simulink library "mbd_s32k1xx_ec_toolbox"  (Simulink 9.0)
settings: Solver=FixedStepDiscrete  StartTime=0.0  StopTime=10.0  FixedStep=0.1  RelTol=1e-3  EnableMultiTasking=on
InitFcn:
  | mbd_s32k_consistency_checks(bdroot(gcs));
(part 2 of 8)

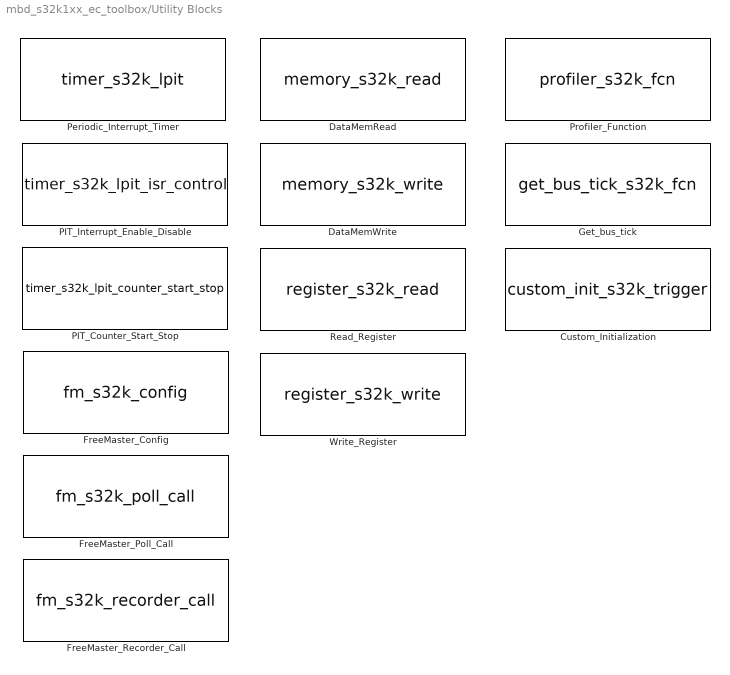
== system mbd_s32k1xx_ec_toolbox/Utility Blocks ==
  Custom_Initialization : S-Function  FunctionName=custom_init_s32k_trigger  SFunctionDeploymentMode=off  EnableBusSupport=off  mask(custom_init_s32k_trigger_block){}
      mask help: This block allows user to insert custom initialization code
      settings: NameChangeFcn=mbd_s12zvc_name_check(gcb);
      mask Help: web(fullfile(mbd_s32k_block_help, 'custom_init', 'custom_init_trigger.html'));
      mask Display:
      | disp('Initialization Call Insertion');
      | port_label('output', 1, 'Trigger');
      | image('nxp_logo.png', 'top-right');
  DataMemRead : S-Function  FunctionName=memory_s32k_read  Parameters=ptr_type  SFunctionDeploymentMode=off  EnableBusSupport=off  mask(memory_s32k_read){base=0x20000000, offset=0x0000, ptr=uint32_t}
      mask prompts: base "Address"; ptr "Pointer type"
      mask help: This block allows a direct memory read from the specified memory location.
      mask init:
      | [maskStr, ptr_type] = mbd_s32k_mem_init();
      settings: NameChangeFcn=mbd_s32k_name_check(gcb);
      mask Help: web(fullfile(mbd_s32k_block_help, 'memory', 'memory_read.html'));
      mask Callback base:
      | str = get_param(gcb, 'base');
      | len = length(str);
      | size = 8;
      | 
      | if (len > 2)
      |     if (strcmp(str(1:2), '0x'))
      |         str = str(3:len);
      |     end
      | end
      | %check if str is a valid hex number. if not, make a valid hex
      | isAllHex = all(isstrprop(str, 'xdigit'));
      | if (~isAllHex)
      |         str = dec2hex(0,size);
      |         len = length(str);
      | end
      | %get address from string
      | value = hex2dec(str);
      | 
      | %check range
      | if (value < 0)
      |     value = 0;
      | elseif (value > hex2dec('FFFF0000'))
      |     value = hex2dec('FFFF0000');
      | end
      | 
      | set_param(gcb, 'base', strcat('0x',dec2hex(value,size)));
      mask Callback offset:
      | str = get_param(gcb, 'offset');
      | len = length(str);
      | size = 4;
      | 
      | if (len > 2)
      |     if (strcmp(str(1:2), '0x'))
      |         str = str(3:len);
      |     end
      | end
      | %check if str is a valid hex number. if not, make a valid hex
      | isAllHex = all(isstrprop(str, 'xdigit'));
      | if (~isAllHex)
      |         str = dec2hex(0,size);
      |         len = length(str);
      | end
      | %get address from string
      | value = hex2dec(str);
      | 
      | %check range
      | if (value < 0)
      |     value = 0;
      | elseif (value > hex2dec('FFFF'))
      |     value = hex2dec('FFFF');
      | end
      | 
      | set_param(gcb, 'offset', strcat('0x',dec2hex(value,size)));
      mask TypeOptions ptr: uint8_t | uint16_t | uint32_t
      mask Display:
      | image('nxp_logo.png', 'top-right');
      | port_label('output',1,'Output');
      | 
      | disp(maskStr);
  DataMemWrite : S-Function  FunctionName=memory_s32k_write  Parameters=ptr_type  SFunctionDeploymentMode=off  EnableBusSupport=off  mask(memory_s32k_write){base=0x20000000, offset=0x0000, ptr=uint32_t}
      mask prompts: base "Address"; ptr "Pointer type"
      mask help: This block allows a direct write to the specified memory location.
      mask init:
      | [maskStr, ptr_type] = mbd_s32k_mem_init();
      settings: NameChangeFcn=mbd_s32k_name_check(gcb);
      mask Help: web(fullfile(mbd_s32k_block_help, 'memory', 'memory_write.html'));
      mask Callback base:
      | str = get_param(gcb, 'base');
      | len = length(str);
      | size = 8;
      | 
      | if (len > 2)
      |     if (strcmp(str(1:2), '0x'))
      |         str = str(3:len);
      |     end
      | end
      | %check if str is a valid hex number. if not, make a valid hex
      | isAllHex = all(isstrprop(str, 'xdigit'));
      | if (~isAllHex)
      |         str = dec2hex(0,size);
      |         len = length(str);
      | end
      | %get address from string
      | value = hex2dec(str);
      | 
      | %check range
      | if (value < 0)
      |     value = 0;
      | elseif (value > hex2dec('FFFF0000'))
      |     value = hex2dec('FFFF0000');
      | end
      | 
      | set_param(gcb, 'base', strcat('0x',dec2hex(value,size)));
      mask Callback offset:
      | str = get_param(gcb, 'offset');
      | len = length(str);
      | size = 4;
      | 
      | if (len > 2)
      |     if (strcmp(str(1:2), '0x'))
      |         str = str(3:len);
      |     end
      | end
      | %check if str is a valid hex number. if not, make a valid hex
      | isAllHex = all(isstrprop(str, 'xdigit'));
      | if (~isAllHex)
      |         str = dec2hex(0,size);
      |         len = length(str);
      | end
      | %get address from string
      | value = hex2dec(str);
      | 
      | %check range
      | if (value < 0)
      |     value = 0;
      | elseif (value > hex2dec('FFFF'))
      |     value = hex2dec('FFFF');
      | end
      | 
      | set_param(gcb, 'offset', strcat('0x',dec2hex(value,size)));
      mask TypeOptions ptr: uint8_t | uint16_t | uint32_t
      mask Display:
      | image('nxp_logo.png', 'top-right');
      | port_label('input',1,'Input');
      | 
      | disp(maskStr);
  FreeMaster_Config : S-Function  FunctionName=fm_s32k_config  Parameters=sFuncParams  SFunctionDeploymentMode=off  EnableBusSupport=off  mask(fm_s32k_config){interface=LPUART1, baudrate=19200, rxd=PTC6: [LPUART1_RX | Receive], txd=PTC7: [LPUART1_TX | Transmit], mode=Poll-driven, isr_prio=15, show_adv_opts=off, use_scope=on, max_scope_vars=8, use_recorder=on, max_rec_vars=8, rec_buff_size=1024, rec_timebase=0, rec_timebase_unit=seconds, comm_buffer_size_auto=on, comm_buffer_size=255, comm_rqueue_size_default=on, comm_rqueue_size=32}
      mask prompts: baudrate "Baud Rate"; rxd "RxD pin"; txd "TxD pin"; isr_prio "ISR Priority"; show_adv_opts "Show Advanced Options"; use_scope "Use Scope"; max_scope_vars "Max Variables"; use_recorder "Use Reccorder"; max_rec_vars "Max Variables"; rec_buff_size "Buffer size (0 - 65536)"; rec_timebase "Timebase (0 - 16384)"; comm_buffer_size_auto "Automatic buffer size"; comm_buffer_size "Buffer size (1-255)"; comm_rqueue_size_default "Default FIFO receiver queue size"; comm_rqueue_size "FIFO receiver queue size (1 - 255)"
      mask help: This block allows the user to configure the FreeMaster embedded-side software driver.
      mask init:
      | mbd_s32k_fm_config_init;
      | mbd_s32k_fm_display_instances;
      settings: NameChangeFcn=mbd_s32k_name_check(gcb);
      mask Help: web(fullfile(mbd_s32k_block_help, 'fm', 'fm_config.html'));
      mask TypeOptions interface: LPUART0 | LPUART1 | LPUART2 | CAN0 | CAN1 | CAN2
      mask Callback interface:
      | mbd_s32k_fm_config_cbk('interface');
      | mbd_s32k_fm_display_instances();
      mask TypeOptions baudrate: 1200 | 2400 | 4800 | 9600 | 14400 | 19200 | 38400 | 56000 | 57600 | 115200 | 128000 | 256000
      mask TypeOptions rxd: PTA19: [LPUART1_RX | Receive] | PTB23: [LPUART1_RX | Receive] | PTC6: [LPUART1_RX | Receive] | PTC8: [LPUART1_RX | Receive] | PTD13: [LPUART1_RX | Receive]
      mask TypeOptions txd: PTA18: [LPUART1_TX | Transmit] | PTB22: [LPUART1_TX | Transmit] | PTC7: [LPUART1_TX | Transmit] | PTC9: [LPUART1_TX | Transmit] | PTD14: [LPUART1_TX | Transmit]
      mask TypeOptions mode: Long Interrupt | Short Interrupt | Poll-driven
      mask Callback mode: mbd_s32k_fm_config_cbk('mode')
      mask TypeOptions isr_prio: 0 | 1 | 2 | 3 | 4 | 5 | 6 | 7 | 8 | 9 | 10 | 11 | 12 | 13 | 14 | 15
      mask Callback show_adv_opts: mbd_s32k_fm_config_cbk('show_adv_opts')
      mask Callback use_scope: mbd_s32k_fm_config_cbk('use_scope')
      mask TypeOptions max_scope_vars: 2 | 3 | 4 | 5 | 6 | 7 | 8
      mask Callback use_recorder: mbd_s32k_fm_config_cbk('use_recorder')
      mask TypeOptions max_rec_vars: 2 | 3 | 4 | 5 | 6 | 7 | 8
      mask TypeOptions rec_timebase_unit: seconds | milliseconds | microseconds | nanoseconds
      mask Callback comm_buffer_size_auto: mbd_s32k_fm_config_cbk('comm_buffer_size_auto')
      mask Callback comm_rqueue_size_default: mbd_s32k_fm_config_cbk('comm_rqueue_size_default')
      mask Display:
      | image('nxp_logo.png', 'top-right');
      | disp(maskStr)
  FreeMaster_Poll_Call : S-Function  FunctionName=fm_s32k_poll_call  SFunctionDeploymentMode=off  EnableBusSupport=off  mask(fm_s32k_poll_call){}
      mask help: This block allows the user to call the FMSTR_Call function in other places then main loop. The FMSTR_Call is placed in the main application loop when this block is not used.
      settings: NameChangeFcn=mbd_s32k_name_check(gcb);
      mask Help: web(fullfile(mbd_s32k_block_help, 'fm', 'fm_poll_call.html'));
      mask Display:
      | image('nxp_logo.png', 'top-right');
      | disp('FreeMaster Poll Call')
  FreeMaster_Recorder_Call : S-Function  FunctionName=fm_s32k_recorder_call  SFunctionDeploymentMode=off  EnableBusSupport=off  mask(fm_s32k_recorder_call){}
      mask help: This block allows the user to call the FMSTR_Recorder function periodically, in places where the data recording should occur.
      settings: NameChangeFcn=mbd_s32k_name_check(gcb);
      mask Help: web(fullfile(mbd_s32k_block_help, 'fm', 'fm_recorder_call.html'));
      mask Display:
      | image('nxp_logo.png', 'top-right');
      | disp('FreeMaster Recorder Call')
  Get_bus_tick : S-Function  FunctionName=get_bus_tick_s32k_fcn  SFunctionDeploymentMode=off  EnableBusSupport=off  mask(get_bus_tick_s32k_func){}
      mask help: This block outputs current bus tick count. You can use 2 of these blocks to emulate a profiler block (by subtracting finish - start) in situations where profiler block can't be used.
      settings: NameChangeFcn=mbd_s32k_name_check(gcb);
      mask Help: web(fullfile(mbd_s32k_block_help, 'profiler', 'get_bus_tick.html'));
      mask Display:
      | port_label('output', 1, 'Bus tick');
      | disp('Get current\n bus tick number');
      | image('nxp_logo.png', 'top-right');
  PIT_Counter_Start_Stop : S-Function  FunctionName=timer_s32k_lpit_counter_start_stop  SFunctionDeploymentMode=off  EnableBusSupport=off  mask(timer_s32k_lpit_counter_start_stop){channel=0, action=Start}
      mask prompts: channel "PIT channel"
      mask help: This block starts or stops the timer channel for PIT block.
      mask init:
      | maskStr = mbd_s32k_lpit_start_stop_init();
      settings: NameChangeFcn=mbd_s32k_name_check(gcb);
      mask Help: web(fullfile(mbd_s32k_block_help, 'lpit', 'timer_lpit_counter_start_stop.html'));
      mask TypeOptions channel: 0 | 1 | 2 | 3
      mask TypeOptions action: Start | Stop
      mask Display:
      | disp(maskStr);
      | image('nxp_logo.png', 'top-right');
  PIT_Interrupt_Enable_Disable : S-Function  FunctionName=timer_s32k_lpit_isr_control  SFunctionDeploymentMode=off  EnableBusSupport=off  mask(timer_s32k_lpit_isr_control){channel=0, enable=off}
      mask prompts: channel "PIT channel"; enable "Enable Timer Interrupt"
      mask help: This block enables or disables the interrupt for PIT block.
      mask init:
      | maskStr = mbd_s32k_lpit_disen_init();
      settings: NameChangeFcn=mbd_s32k_name_check(gcb);
      mask Help: web(fullfile(mbd_s32k_block_help, 'lpit', 'timer_lpit_isr_control.html'));
      mask TypeOptions channel: 0 | 1 | 2 | 3
      mask Display:
      | disp(maskStr);
      | image('nxp_logo.png', 'top-right');
  Periodic_Interrupt_Timer : S-Function  FunctionName=timer_s32k_lpit  SFunctionDeploymentMode=off  EnableBusSupport=off  mask(timer_s32k_lpit){channel=0, period=500000, prio=15, startCounter=on}
      mask prompts: channel "PIT Channel"; period "Period Value (us)"; prio "ISR Priority"; startCounter "Start counter immediately after initialization"
      mask help: This block triggers an interrupt routine to execute every timeout of this LPIT channel in 32-bit Periodic Counter Mode.
      mask init:
      | maskStr = mbd_s32k_lpit_init();
      settings: NameChangeFcn=mbd_s32k_name_check(gcb);
      mask Help: web(fullfile(mbd_s32k_block_help, 'lpit', 'timer_pit.html'));
      mask TypeOptions channel: 0 | 1 | 2 | 3
      mask TypeOptions prio: 0 | 1 | 2 | 3 | 4 | 5 | 6 | 7 | 8 | 9 | 10 | 11 | 12 | 13 | 14 | 15
      mask Callback prio: mbd_s32k_isr_priority_cbk(gcb, 'prio');
      mask Display:
      | disp(maskStr);
      | port_label('output',1,'trigger');
      | image('nxp_logo.png', 'top-right');
  Profiler_Function : S-Function  FunctionName=profiler_s32k_fcn  Parameters=profile_indx, showOut  SFunctionDeploymentMode=off  EnableBusSupport=off  mask(profiler_s32k_func){profile_indx=0, showOut=on}
      mask prompts: profile_indx "Select the profile Index"; showOut "Show Profile Output"
      mask help: Place this block inside a subsystem (even top level) in order to profile it. You can profile up to 100 different subsystems with this block, as long as you make sure to select a different profile index for each one.
      settings: NameChangeFcn=mbd_s32k_name_check(gcb);
      mask Help: web(fullfile(mbd_s32k_block_help, 'profiler', 'profiler_function.html'));
      mask TypeOptions profile_indx: 0 | 1 | 2 | 3 | 4 | 5 | 6 | 7 | 8 | 9 | 10 | 11 | 12 | 13 | 14 | 15 | 16 | 17 | 18 | 19 | 20 | 21 | 22 | 23 | 24 | 25 | 26 | 27 | 28 | 29 | 30 | 31 | 32 | 33 | 34 | 35 | 36 | 37 | 38 | 39 | 40 | 41 | 42 | 43 | 44 | 45 | 46 | 47 | 48 | 49 | 50 | 51 | 52 | 53 | 54 | 55 | 56 | 57 | 58 | 59 | 60 | 61 | 62 | 63 | 64 | 65 | 66 | 67 | 68 | 69 | 70 | 71 | 72 | 73 | 74 | 75 | 76 | 77 | 78 | 79 | 80 | 81 | 82 | 83 | 84 | 85 | 86 | 87 | 88 | 89 | 90 | 91 | 92 | 93 | 94 | 95 | 96 | 97 | 98 | 99
      mask Display:
      | disp(['Profile Function Index : ',get_param(gcb,'profile_indx')]);
      | image('nxp_logo.png', 'top-right');
  Read_Register : S-Function  FunctionName=register_s32k_read  Parameters=index  SFunctionDeploymentMode=off  EnableBusSupport=off  mask(register_s32k_read){periph=ADC0, reg=SC1A, addr=0x4003B000, regSize=32, pcc_clock=ADC0_CLK}
      mask prompts: periph "Peripheral"; reg "Register"; addr "Address"; regSize "Size (bits)"; pcc_clock "PCC clock"
      mask help: This block allows direct access to read a register.
      mask init:
      | mbd_s32k_rw_register_init;
      mask Help: web(fullfile(mbd_s32k_block_help, 'reg', 'read_register.html'));
      mask TypeOptions periph: ADC0 | ADC1 | AIPS | CAN0 | CAN1 | CAN2 | CMP0 | CRC | CSE_PRAM | DMA | DMAMUX | EIM | ENET | ERM | EWM | FLEXIO | FTFC | FTM0 | FTM1 | FTM2 | FTM3 | FTM4 | FTM5 | FTM6 | FTM7 | LMEM | LPI2C0 | LPI2C1 | LPIT0 | LPSPI0 | LPSPI1 | LPSPI2 | LPTMR0 | LPUART0 | LPUART1 | LPUART2 | MCM | MPU | MSCM | PCC | PDB0 | PDB1 | PMC | PORTA | PORTB | PORTC | PORTD | PORTE | PTA | PTB | PTC | PTD | PTE | Qu | RCM | RTC | S32_NVIC | S32_SCB | S32_SysTick | SAI0 | SAI1 | SCG | SIM | SMC | TRGMUX | WDOG
      mask Callback periph: mbd_s32k_periph_update_cbk('read');
      mask TypeOptions reg: SC1A | SC1B | SC1C | SC1D | SC1E | SC1F | SC1G | SC1H | SC1I | SC1J | SC1K | SC1L | SC1M | SC1N | SC1O | SC1P | CFG1 | CFG2 | RA | RB | RC | RD | RE | RF | RG | RH | RI | RJ | RK | RL | RM | RN | RO | RP | CV1 | CV2 | SC2 | SC3 | BASE_OFS | OFS | USR_OFS | XOFS | YOFS | G | UG | CLPS | CLP3 | CLP2 | CLP1 | CLP0 | CLPX | CLP9 | CLPS_OFS | CLP3_OFS | CLP2_OFS | CLP1_OFS | CLP0_OFS | CLPX_OFS | CLP9_OFS | aSC1A | aSC1B | aSC1C | aSC1D | aSC1E | aSC1F | aSC1G | aSC1H | aSC1I | aSC1J | aSC1K | aSC1L | aSC1M | aSC1N | aSC1O | aSC1P | SC1Q | SC1R | SC1S | SC1T | SC1U | SC1V | SC1W | SC1X | SC1Y | SC1Z | SC1AA | SC1AB | SC1AC | SC1AD | SC1AE | SC1AF | aRA | aRB | aRC | aRD | aRE | aRF | aRG | aRH | aRI | aRJ | aRK | aRL | aRM | aRN | aRO | aRP | RQ | RR | RS | RT | RU | RV | RW | RX | RY | RZ | RAA | RAB | RAC | RAD | RAE | RAF
      mask Callback reg: mbd_s32k_reg_update_cbk;
      mask DialogControl descript Prompt: ADC Status and Control Register 1
      mask Display:
      | image('nxp_logo.png', 'top-right');
      | port_label('output',1,'Output');
      | disp(maskStr);
  Write_Register : S-Function  FunctionName=register_s32k_write  Parameters=index  SFunctionDeploymentMode=off  EnableBusSupport=off  mask(register_s32k_write){periph=ADC0, reg=SC1A, addr=0x4003B000, regsize=32, pcc_clock=ADC0_CLK}
      mask prompts: periph "Peripheral"; reg "Register"; addr "Address"; regsize "Size (bits)"; pcc_clock "PCC clock"
      mask help: This block allows direct access to write a register
      mask init:
      | mbd_s32k_rw_register_init;
      mask Help: web(fullfile(mbd_s32k_block_help, 'reg', 'write_register.html'));
      mask TypeOptions periph: ADC0 | ADC1 | AIPS | CAN0 | CAN1 | CAN2 | CMP0 | CRC | CSE_PRAM | DMA | DMAMUX | EIM | ENET | ERM | EWM | FLEXIO | FTFC | FTM0 | FTM1 | FTM2 | FTM3 | FTM4 | FTM5 | FTM6 | FTM7 | LMEM | LPI2C0 | LPI2C1 | LPIT0 | LPSPI0 | LPSPI1 | LPSPI2 | LPTMR0 | LPUART0 | LPUART1 | LPUART2 | MCM | MPU | MSCM | PCC | PDB0 | PDB1 | PMC | PORTA | PORTB | PORTC | PORTD | PORTE | PTA | PTB | PTC | PTD | PTE | Qu | RCM | RTC | S32_NVIC | S32_SCB | S32_SysTick | SAI0 | SAI1 | SCG | SIM | SMC | TRGMUX | WDOG
      mask Callback periph: mbd_s32k_periph_update_cbk('write')
      mask TypeOptions reg: SC1A | SC1B | SC1C | SC1D | SC1E | SC1F | SC1G | SC1H | SC1I | SC1J | SC1K | SC1L | SC1M | SC1N | SC1O | SC1P | CFG1 | CFG2 | CV1 | CV2 | SC2 | SC3 | BASE_OFS | OFS | USR_OFS | XOFS | YOFS | G | UG | CLPS | CLP3 | CLP2 | CLP1 | CLP0 | CLPX | CLP9 | CLPS_OFS | CLP3_OFS | CLP2_OFS | CLP1_OFS | CLP0_OFS | CLPX_OFS | CLP9_OFS | aSC1A | aSC1B | aSC1C | aSC1D | aSC1E | aSC1F | aSC1G | aSC1H | aSC1I | aSC1J | aSC1K | aSC1L | aSC1M | aSC1N | aSC1O | aSC1P | SC1Q | SC1R | SC1S | SC1T | SC1U | SC1V | SC1W | SC1X | SC1Y | SC1Z | SC1AA | SC1AB | SC1AC | SC1AD | SC1AE | SC1AF
      mask Callback reg: mbd_s32k_reg_update_cbk;
      mask DialogControl descript Prompt: ADC Status and Control Register 1
      mask Display:
      | image('nxp_logo.png', 'top-right');
      | port_label('input',1,'Input ');
      | disp(maskStr);

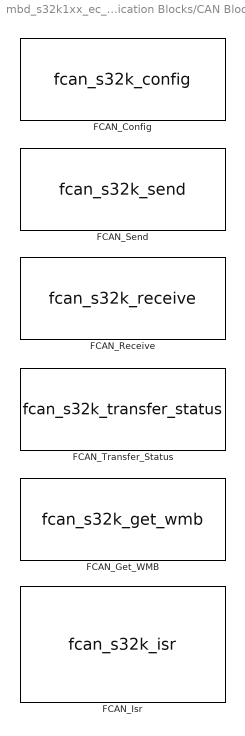
== system mbd_s32k1xx_ec_toolbox/Communication Blocks/CAN Blocks ==
  FCAN_Config : S-Function  FunctionName=fcan_s32k_config  SFunctionDeploymentMode=off  EnableBusSupport=off  mask(fcan_s32k_config){can_instance=0, can_mode=Normal mode, can_max_num_mb=0, can_rx=PTE4: [CAN0_RX | CAN Rx channel], can_tx=PTE5: [CAN0_TX | CAN Tx Channel], show_adv_opts=off, can_clk_src=Peripheral clock, bitrate=500, bitrate_adv_opts=off, can_presdiv=7, can_rjw=3, can_pseg1=6, can_pseg2=3, can_propseg=7, can_cbt_presdiv=3, can_cbt_rjw=3, can_cbt_pseg1=7, can_cbt_pseg2=7, can_cbt_propseg=6, can_fd_enable=off, can_payload=8, can_rxfifo_enable=off, can_fifo_id_filter_extended=off, can_fifo_id_filter_remote=off, can_num_id_filters=8, can_fifo_id_format=A, can_fifo_id_filter={'0x0', '0x0', '0x0', '0x0', '0x0', '0x0', '0x0', '0x0'}, can_pn_enable=off, can_wakeup_match=off, can_wakeup_timeout=off, can_timeout_en=off, can_match_timeout=1, can_multiple_matches_en=off, can_num_matches=1, can_idfilter_extendedid=off, can_idfilter_remoteframe=off, can_idfilter_type=Match exact, can_idfilter_id1=0, can_idfilter_id2=0, can_payloadfilter_enable=off, can_payloadfilter_dlclow=0, can_payloadfilter_dlchigh=0, can_payloadfilter_type=Match exact, can_payloadfilter_payload1_b0=0, can_payloadfilter_payload1_b1=0, can_payloadfilter_payload1_b2=0, can_payloadfilter_payload1_b3=0, can_payloadfilter_payload1_b4=0, can_payloadfilter_payload1_b5=0, can_payloadfilter_payload1_b6=0, can_payloadfilter_payload1_b7=0, can_payloadfilter_payload2_b0=0, can_payloadfilter_payload2_b1=0, can_payloadfilter_payload2_b2=0, can_payloadfilter_payload2_b3=0, can_payloadfilter_payload2_b4=0, can_payloadfilter_payload2_b5=0, can_payloadfilter_payload2_b6=0, can_payloadfilter_payload2_b7=0}
      mask prompts: can_instance "CAN Bus"; can_mode "Operational Mode"; can_max_num_mb "Max number of MBs (0 - 32)"; can_rx "Rx:"; can_tx "Tx:"; show_adv_opts "Show advanced options"; can_clk_src "CAN Engine Clock Source"; bitrate "Bitrate(Kbit/s)"; bitrate_adv_opts "Advanced options"; can_presdiv "Prescaler Divider (0-255)"; can_rjw "Resync Jump Width"; can_pseg1 "Phase Segment 1"; can_pseg2 "Phase Segment 2"; can_propseg "Propagation Segment"; can_cbt_presdiv "Prescaler Divider (0-1023)"; can_cbt_rjw "Resync Jump Width"; can_cbt_pseg1 "Phase Segment 1"; can_cbt_pseg2 "Phase Segment 2"; can_cbt_propseg "Propagation Segment"; can_fd_enable "Enable CAN FD"; can_payload "Payload size"; can_rxfifo_enable "Enable Rx FIFO"; can_fifo_id_filter_extended "Extended ID"; can_fifo_id_filter_remote "Remote frame"; can_num_id_filters "Num ID filters"; can_fifo_id_format "ID format"; can_fifo_id_filter "Filter table"; can_pn_enable "Enable Pretended Networking"; can_wakeup_match "Match event"; can_wakeup_timeout "Timeout event"; can_timeout_en "Enable timeout"; can_match_timeout "Timeout (1 - 65535)"; can_multiple_matches_en "Enable multiple matches"; can_num_matches "Needed matches (1 - 255)"; can_idfilter_extendedid "Extended ID"; can_idfilter_remoteframe "Remote frame"; can_idfilter_type "ID filter type"; can_idfilter_id1 "ID value"; can_idfilter_id2 "ID mask"; can_payloadfilter_enable "Enable payload filtering"; can_payloadfilter_dlclow "Min payload size (0 - 8)"; can_payloadfilter_dlchigh "Max payload size (0 - 8)"; can_payloadfilter_type "Payload filter type"; can_payloadfilter_payload1_b0 "B0"; can_payloadfilter_payload1_b1 "B1"; can_payloadfilter_payload1_b2 "B2"; can_payloadfilter_payload1_b3 "B3"; can_payloadfilter_payload1_b4 "B4"; can_payloadfilter_payload1_b5 "B5"; can_payloadfilter_payload1_b6 "B6"; can_payloadfilter_payload1_b7 "B7"; can_payloadfilter_payload2_b0 "B0"; can_payloadfilter_payload2_b1 "B1"; can_payloadfilter_payload2_b2 "B2"; can_payloadfilter_payload2_b3 "B3"; can_payloadfilter_payload2_b4 "B4"; can_payloadfilter_payload2_b5 "B5"; can_payloadfilter_payload2_b6 "B6"; can_payloadfilter_payload2_b7 "B7"
      mask help: This block is allow to configure FlexCAN module.
      mask init:
      | mbd_s32k_fcan_config_init;
      settings: NameChangeFcn=mbd_s32k_name_check (gcb);
      mask Help: web(fullfile(mbd_s32k_block_help, 'fcan', 'fcan_config.html'));
      mask TypeOptions can_instance: 0 | 1 | 2
      mask Callback can_instance:
      | mbd_s32k_fcan_config_cbk('can_instance');
      | mbd_s32k_fcan_display_instances();
      mask TypeOptions can_mode: Normal mode | Listen-only mode | Loop-back mode
      mask Callback can_max_num_mb: mbd_s32k_fcan_config_cbk('can_max_num_mb');
      mask TypeOptions can_rx: PTA28: [CAN0_RX | CAN Rx channel] | PTB0: [CAN0_RX | CAN Rx channel] | PTC2: [CAN0_RX | CAN Rx channel] | PTE4: [CAN0_RX | CAN Rx channel]
      mask TypeOptions can_tx: PTA27: [CAN0_TX | CAN Tx Channel] | PTB1: [CAN0_TX | CAN Tx Channel] | PTC3: [CAN0_TX | CAN Tx Channel] | PTE5: [CAN0_TX | CAN Tx Channel]
      mask Callback show_adv_opts: mbd_s32k_fcan_config_cbk('show_adv_opts');
      mask TypeOptions can_clk_src: Oscillator clock | Peripheral clock
      mask Callback can_clk_src: mbd_s32k_fcan_config_cbk('can_clk_src')
      mask TypeOptions bitrate: 50 | 100 | 125 | 250 | 500 | 1000
      mask Callback bitrate: mbd_s32k_fcan_config_cbk('bitrate')
      mask Callback bitrate_adv_opts: mbd_s32k_fcan_config_cbk('bitrate_adv_opts')
      mask TypeOptions can_rjw: 0 | 1 | 2 | 3
      mask TypeOptions can_pseg1: 0 | 1 | 2 | 3 | 4 | 5 | 6 | 7
      mask TypeOptions can_pseg2: 1 | 2 | 3 | 4 | 5 | 6 | 7
      mask TypeOptions can_propseg: 0 | 1 | 2 | 3 | 4 | 5 | 6 | 7
      mask TypeOptions can_cbt_rjw: 0 | 1 | 2 | 3
      mask TypeOptions can_cbt_pseg1: 0 | 1 | 2 | 3 | 4 | 5 | 6 | 7
      mask TypeOptions can_cbt_pseg2: 1 | 2 | 3 | 4 | 5 | 6 | 7
      mask TypeOptions can_cbt_propseg: 0 | 1 | 2 | 3 | 4 | 5 | 6 | 7 | 8 | 9 | 10 | 11 | 12 | 13 | 14 | 15 | 16 | 17 | 18 | 19 | 20 | 21 | 22 | 23 | 24 | 25 | 26 | 27 | 28 | 29 | 30 | 31
      mask Callback can_fd_enable: mbd_s32k_fcan_config_cbk('can_fd_enable');
      mask TypeOptions can_payload: 8
      mask Callback can_rxfifo_enable: mbd_s32k_fcan_config_cbk('can_rxfifo_enable');
      mask TypeOptions can_num_id_filters: 8 | 16 | 24 | 32 | 40 | 48 | 56 | 64 | 72 | 80 | 88 | 96 | 104 | 112 | 120 | 128
      mask TypeOptions can_fifo_id_format: A | B | C | D
      mask Callback can_pn_enable: mbd_s32k_fcan_config_cbk('can_pn_enable');
      mask Callback can_timeout_en: mbd_s32k_fcan_config_cbk('can_timeout_en');
      mask Callback can_multiple_matches_en: mbd_s32k_fcan_config_cbk('can_multiple_matches_en');
      mask TypeOptions can_idfilter_type: Match exact | Match greater than or equal to | Match less than or equal to | Match in range
      mask Callback can_payloadfilter_enable: mbd_s32k_fcan_config_cbk('can_payloadfilter_enable');
      mask TypeOptions can_payloadfilter_type: Match exact | Match greater than or equal to | Match less than or equal to | Match in range
      mask DialogControl PinsGroupbox Prompt: Pins
      mask DialogControl CanStandardFrameGroupbox Prompt: CAN Standard Frame
      mask DialogControl ArbitrationPhaseGroupbox Prompt: Arbitration Phase
      mask DialogControl DataPhaseGroupbox Prompt: Data Phase
      mask DialogControl RxFifoFilteringGroupbox Prompt: Rx FIFO Filtering
      mask DialogControl WakeUpEventsGroupbox Prompt: Wake Up Events
      mask DialogControl IdFilteringGroupbox Prompt: ID Filtering
      mask DialogControl PayloadFilteringGroupbox Prompt: Payload Filtering
      mask DialogControl PayloadValueGroupbox Prompt: Payload value
      mask DialogControl PayloadMaskGroupbox Prompt: Payload mask
      mask Display:
      | image('nxp_logo.png', 'top-right');
      | disp(st);
  FCAN_Get_WMB : S-Function  FunctionName=fcan_s32k_get_wmb  SFunctionDeploymentMode=off  EnableBusSupport=off  mask(fcan_s32k_get_wmb){can_instance=0, can_wmb_idx=0}
      mask prompts: can_instance "CAN Bus"; can_wmb_idx "Wake up Message Buffer"
      mask help: This block allows user to get the Rx data received when FlexCAN is in Pretended Networking mode.
      mask init:
      | crlf = sprintf('\n');
      | 
      | st = [
      |     'FCAN Module : ' get_param(gcb, 'can_instance') crlf ...
      |     'Wake up Message Buffer : ' get_param(gcb, 'can_wmb_idx') crlf];
      settings: NameChangeFcn=mbd_s32k_name_check (gcb);
      mask Help: web(fullfile(mbd_s32k_block_help, 'fcan', 'fcan_get_wmb.html'));
      mask TypeOptions can_instance: 0
      mask TypeOptions can_wmb_idx: 0 | 1 | 2 | 3
      mask Display:
      | image('nxp_logo.png', 'top-right');
      | disp(st);
      | 
      | port_label('output', 1, 'ID');
      | port_label('output', 2, 'Data');
      | port_label('output', 3, 'Length');
  FCAN_Isr : S-Function  FunctionName=fcan_s32k_isr  Parameters=sFuncParams  SFunctionDeploymentMode=off  EnableBusSupport=off  mask(fcan_s32k_isr){can_instance=0, can_event=Rx Complete}
      mask prompts: can_instance "CAN Bus"; can_event "Event"
      mask help: This block allows to call user function on different FlexCAN events.
      mask init:
      | [maskStr, sFuncParams] = mbd_s32k_fcan_isr();
      settings: NameChangeFcn=mbd_s32k_name_check (gcb);
      mask Help: web(fullfile(mbd_s32k_block_help, 'fcan', 'fcan_isr.html'));
      mask TypeOptions can_instance: 0 | 1 | 2
      mask Callback can_instance:
      | mbd_s32k_fcan_isr_cbk('can_instance');
      | mbd_s32k_fcan_display_instances();
      mask TypeOptions can_event: Rx Complete | Rx FIFO Complete | Tx Complete | Wake Up Timeout | Wake Up Match | Rx FIFO Warning | Rx FIFO Overflow
      mask Display:
      | image('nxp_logo.png', 'top-right');
      | disp(maskStr);
      | 
      | event = get_param(gcb, 'can_event');
      | 
      | rxCompleteEvent = strcmp(event, 'Rx Complete');
      | rxFifoCompleteEvent = strcmp(event, 'Rx FIFO Complete');
      | txComplete = strcmp(event, 'Tx Complete');
      | 
      | port_label('output', 1, 'Trigger');
      | 
      | switch event
      |     case 'Rx Complete'
      |         port_label('output', 2, 'MB Index');
      |         port_label('output', 3, 'ID');
      |         port_label('output', 4, 'Data');
      |         port_label('output', 5, 'Length');
      |         port_label('output', 6, 'Timestamp');
      |     case 'Rx FIFO Complete'
      |         port_label('output', 2, 'ID');
      |         port_label('output', 3, 'Data');
      |         port_label('output', 4, 'Length');
      |         port_label('output', 5, 'Timestamp');
      |     case 'Tx Complete'
      |         port_label('output', 2, 'MB Index');
      |     case 'Rx FIFO Warning'
      |         port_label('output', 2, 'MB Index');
      |     case 'Rx FIFO Overflow'
      |         port_label('output', 2, 'MB Index');
      | end
  FCAN_Receive : S-Function  FunctionName=fcan_s32k_receive  Parameters=sFuncParams  SFunctionDeploymentMode=off  EnableBusSupport=off  mask(fcan_s32k_receive){can_instance=0, can_mode=Non-blocking, can_timeout_ms=0, can_mb_idx=0, can_extended_id=off, can_is_remote=off, can_id=0, can_msg_mask=0, show_adv_opts=off, can_use_rxfifo=off, can_fd_enable=off}
      mask prompts: can_instance "CAN Bus"; can_mode "Mode"; can_timeout_ms "Timeout (ms)"; can_mb_idx "Message Buffer"; can_extended_id "Extended ID"; can_is_remote "Remote message"; can_id "ID (0 - 0x7FF)"; can_msg_mask "Message ID mask (0 - 0xFFFFFFFF)"; show_adv_opts "Show advanced options"; can_use_rxfifo "Use Rx FIFO"; can_fd_enable "Enable CAN FD"
      mask help: This block allows the user to receive data throught CAN interface.
      mask init:
      | [maskStr sFuncParams] = mbd_s32k_fcan_receive();
      settings: NameChangeFcn=mbd_s32k_name_check (gcb);
      mask Help: web(fullfile(mbd_s32k_block_help, 'fcan', 'fcan_receive.html'));
      mask TypeOptions can_instance: 0 | 1 | 2
      mask Callback can_instance: mbd_s32k_fcan_receive_cbk('can_instance');
      mask TypeOptions can_mode: Blocking | Non-blocking
      mask Callback can_mode: mbd_s32k_fcan_receive_cbk('can_mode');
      mask TypeOptions can_mb_idx: 0 | 1 | 2 | 3 | 4 | 5 | 6 | 7 | 8 | 9 | 10 | 11 | 12 | 13 | 14 | 15 | 16 | 17 | 18 | 19 | 20 | 21 | 22 | 23 | 24 | 25 | 26 | 27 | 28 | 29 | 30 | 31
      mask Callback can_extended_id: mbd_s32k_fcan_receive_cbk('can_extended_id');
      mask Callback can_id: mbd_s32k_fcan_receive_cbk('can_id');
      mask Callback can_msg_mask: mbd_s32k_fcan_receive_cbk('can_msg_mask');
      mask Callback show_adv_opts: mbd_s32k_fcan_receive_cbk('show_adv_opts');
      mask Callback can_use_rxfifo: mbd_s32k_fcan_receive_cbk('can_use_rxfifo');
      mask Callback can_fd_enable: mbd_s32k_fcan_receive_cbk('can_fd_enable');
      mask DialogControl MailboxGroupbox Prompt: Mailbox
      mask Display:
      | image('nxp_logo.png', 'top-right');
      | disp(maskStr);
      | 
      | mode = get_param(gcb, 'can_mode');
      | if strcmp(mode, 'Blocking')
      |     port_label('output', 1, 'Status');
      |     port_label('output', 2, 'ID');
      |     port_label('output', 3, 'Data');
      |     port_label('output', 4, 'Length');
      |     port_label('output', 5, 'Timestamp');
      | end
  FCAN_Send : S-Function  FunctionName=fcan_s32k_send  Parameters=out  SFunctionDeploymentMode=off  EnableBusSupport=off  mask(fcan_s32k_send){can_instance=0, can_mode=Non-blocking, can_timeout_ms=0, can_mb_idx=0, can_extended_id=off, can_is_remote=off, can_id=0, show_adv_opts=off, can_fd_enable=off, can_enable_brs=off, can_fd_padding=0}
      mask prompts: can_instance "CAN Bus"; can_mode "Mode"; can_timeout_ms "Timeout (ms)"; can_mb_idx "Message Buffer"; can_extended_id "Extended ID"; can_is_remote "Remote message"; can_id "ID (0 - 0x7FF)"; show_adv_opts "Show advanced options"; can_fd_enable "Enable CAN FD"; can_enable_brs "Enable Bit Rate Switch (BRS)"; can_fd_padding "CAN FD Padding (0 - 0xFF)"
      mask help: This block allows user to send data throught CAN interface.
      mask init:
      | mbd_s32k_fcan_send_init;
      settings: NameChangeFcn=mbd_s32k_name_check (gcb);
      mask Help: web(fullfile(mbd_s32k_block_help, 'fcan', 'fcan_send.html'));
      mask TypeOptions can_instance: 0 | 1 | 2
      mask Callback can_instance: mbd_s32k_fcan_send_cbk('can_instance');
      mask TypeOptions can_mode: Blocking | Non-blocking
      mask Callback can_mode: mbd_s32k_fcan_send_cbk('can_mode');
      mask TypeOptions can_mb_idx: 0 | 1 | 2 | 3 | 4 | 5 | 6 | 7 | 8 | 9 | 10 | 11 | 12 | 13 | 14 | 15 | 16 | 17 | 18 | 19 | 20 | 21 | 22 | 23 | 24 | 25 | 26 | 27 | 28 | 29 | 30 | 31
      mask Callback can_extended_id: mbd_s32k_fcan_send_cbk('can_extended_id');
      mask Callback can_id: mbd_s32k_fcan_send_cbk('can_id');
      mask Callback show_adv_opts: mbd_s32k_fcan_send_cbk('show_adv_opts');
      mask Callback can_fd_enable: mbd_s32k_fcan_send_cbk('can_fd_enable');
      mask Callback can_fd_padding: mbd_s32k_fcan_send_cbk('can_fd_padding');
      mask DialogControl MailboxGroupbox Prompt: Mailbox
      mask DialogControl CanFdGroupbox Prompt: CAN FD
      mask Display:
      | image('nxp_logo.png', 'top-right');
      | disp(st);
      | 
      | port_label('input', 1, 'Data');
      | port_label('input', 2, 'Length');
      | 
      | mode = get_param(gcb, 'can_mode');
      | if strcmp(mode, 'Blocking')
      |     port_label('output', 1, 'Status');
      | end
  FCAN_Transfer_Status : S-Function  FunctionName=fcan_s32k_transfer_status  SFunctionDeploymentMode=off  EnableBusSupport=off  mask(fcan_s32k_transfer_status){can_instance=0, can_mb_idx=0}
      mask prompts: can_instance "CAN Bus"; can_mb_idx "Message Buffer"
      mask help: This block allows the user to query if a FlexCAN transfer has finished.
      mask init:
      | mbd_s32k_fcan_transfer_status_init;
      settings: NameChangeFcn=mbd_s32k_name_check (gcb);
      mask Help: web(fullfile(mbd_s32k_block_help, 'fcan', 'fcan_transfer_status.html'));
      mask TypeOptions can_instance: 0 | 1 | 2
      mask Callback can_instance: mbd_s32k_fcan_transfer_status_cbk('can_instance');
      mask TypeOptions can_mb_idx: 0 | 1 | 2 | 3 | 4 | 5 | 6 | 7 | 8 | 9 | 10 | 11 | 12 | 13 | 14 | 15 | 16 | 17 | 18 | 19 | 20 | 21 | 22 | 23 | 24 | 25 | 26 | 27 | 28 | 29 | 30 | 31
      mask Display:
      | image('nxp_logo.png', 'top-right');
      | disp(st);
      | 
      | port_label('output', 1, 'Busy');

== system mbd_s32k1xx_ec_toolbox/Communication Blocks/FlexIO Blocks  ==
  FlexIO I2C Blocks : Subsystem
  FlexIO SPI Blocks : Subsystem
  FlexIO UART Blocks : Subsystem

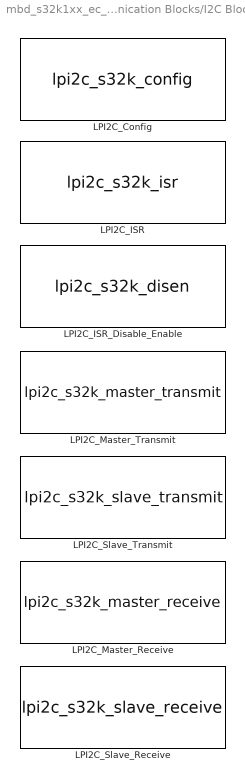
== system mbd_s32k1xx_ec_toolbox/Communication Blocks/I2C Blocks ==
  LPI2C_Config : S-Function  FunctionName=lpi2c_s32k_config  SFunctionDeploymentMode=off  EnableBusSupport=off  mask(lpi2c_s32k_config){instance=0, mode=Master, opmode=Standard (up to 100 kbit/s), bdr=100000, addr=1, is10bitaddr=off, sda=PTA2: [LPI2C0_SDA | LPI2C Data I/O], scl=PTA3: [LPI2C0_SCL | LPI2C Clock I/O]}
      mask prompts: opmode "Operating mode"; bdr "Baudrate, b/s"; addr "null"; is10bitaddr "10-bit address"
      mask help: This block allows to configure I2C module.
      mask init:
      | maskStr = mbd_s32k_lpi2c_config_string();
      | mbd_s32k_lpi2c_display_instances();
      | mbd_s32k_lpi2c_instance_callback(gcb);
      settings: NameChangeFcn=mbd_s32k_name_check(gcb);
      mask Help: web(fullfile(mbd_s32k_block_help, 'lpi2c', 'lpi2c_config.html'));
      mask TypeOptions instance: 0 | 1
      mask Callback instance:
      | mbd_s32k_lpi2c_instance_callback(gcb);
      | mbd_s32k_lpi2c_display_instances();
      mask TypeOptions mode: Master | Slave
      mask Callback mode: mbd_s32k_lpi2c_mode_callback(gcb);
      mask TypeOptions opmode: Standard (up to 100 kbit/s)
      mask Callback bdr: mbd_s32k_lpi2c_check_bdr(gcb);
      mask TypeOptions sda: PTA2: [LPI2C0_SDA | LPI2C Data I/O] | PTB6: [LPI2C0_SDA | LPI2C Data I/O] | PTA1: [LPI2C0_SDAS | LPI2C Secondary Data I/O] | PTA2: [LPI2C0_SDA | LPI2C Data I/O] | PTB6: [LPI2C0_SDA | LPI2C Data I/O] | PTA1: [LPI2C0_SDAS | LPI2C Secondary Data I/O] | PTA2: [LPI2C0_SDA | LPI2C Data I/O] | PTB6: [LPI2C0_SDA | LPI2C Data I/O] | PTA1: [LPI2C0_SDAS | LPI2C Secondary Data I/O] | PTA2: [LPI2C0_SDA | LPI2C Data I/O] | PTB6: [LPI2C0_SDA | LPI2C Data I/O] | PTA1: [LPI2C0_SDAS | LPI2C Secondary Data I/O] | PTA2: [LPI2C0_SDA | LPI2C Data I/O] | PTB6: [LPI2C0_SDA | LPI2C Data I/O] | PTA1: [LPI2C0_SDAS | LPI2C Secondary Data I/O] | PTA2: [LPI2C0_SDA | LPI2C Data I/O] | PTB6: [LPI2C0_SDA | LPI2C Data I/O] | PTA1: [LPI2C0_SDAS | LPI2C Secondary Data I/O] | PTC31: [LPI2C1_SDA | LPI2C Data I/O] | PTD8: [LPI2C1_SDA | LPI2C Data I/O] | PTE0: [LPI2C1_SDA | LPI2C Data I/O] | PTA12: [LPI2C1_SDAS | LPI2C Secondary Data I/O] | PTC16: [LPI2C1_SDAS | LPI2C Secondary Data I/O] | PTC30: [LPI2C1_SDAS | LPI2C Secondary Data I/O]
      mask TypeOptions scl: PTA3: [LPI2C0_SCL | LPI2C Clock I/O] | PTB7: [LPI2C0_SCL | LPI2C Clock I/O] | PTA0: [LPI2C0_SCLS | LPI2C Secondary Clock I/O] | PTA3: [LPI2C0_SCL | LPI2C Clock I/O] | PTB7: [LPI2C0_SCL | LPI2C Clock I/O] | PTA0: [LPI2C0_SCLS | LPI2C Secondary Clock I/O] | PTA3: [LPI2C0_SCL | LPI2C Clock I/O] | PTB7: [LPI2C0_SCL | LPI2C Clock I/O] | PTA0: [LPI2C0_SCLS | LPI2C Secondary Clock I/O] | PTA3: [LPI2C0_SCL | LPI2C Clock I/O] | PTB7: [LPI2C0_SCL | LPI2C Clock I/O] | PTA0: [LPI2C0_SCLS | LPI2C Secondary Clock I/O] | PTA3: [LPI2C0_SCL | LPI2C Clock I/O] | PTB7: [LPI2C0_SCL | LPI2C Clock I/O] | PTA0: [LPI2C0_SCLS | LPI2C Secondary Clock I/O] | PTA3: [LPI2C0_SCL | LPI2C Clock I/O] | PTB7: [LPI2C0_SCL | LPI2C Clock I/O] | PTA0: [LPI2C0_SCLS | LPI2C Secondary Clock I/O] | PTD9: [LPI2C1_SCL | LPI2C Clock I/O] | PTD19: [LPI2C1_SCL | LPI2C Clock I/O] | PTE1: [LPI2C1_SCL | LPI2C Clock I/O] | PTA13: [LPI2C1_SCLS | LPI2C Secondary Clock I/O] | PTC17: [LPI2C1_SCLS | LPI2C Secondary Clock I/O] | PTD18: [LPI2C1_SCLS | LPI2C Secondary Clock I/O]
      mask Display:
      | disp(maskStr);
      | image('nxp_logo.png', 'top-right');
  LPI2C_ISR : S-Function  FunctionName=lpi2c_s32k_isr  SFunctionDeploymentMode=off  EnableBusSupport=off  mask(lpi2c_s32k_isr){instance=0, mode=Master, rxreq=off, txreq=off, txempty=off, rxfull=off, stop=off, masterendtransfer=off, mastertx=off, masterrx=off, masterfifoerr=off, masterarblost=off, masternack=off}
      mask prompts: rxreq "I2C_SLAVE_EVENT_RX_REQ"; txreq "I2C_SLAVE_EVENT_TX_REQ"; txempty "I2C_SLAVE_EVENT_TX_EMPTY"; rxfull "I2C_SLAVE_EVENT_RX_FULL"; stop "I2C_SLAVE_EVENT_STOP"; masterendtransfer "I2C_MASTER_EVENT_END_TRANSFER"; mastertx "LPI2C_MASTER_EVENT_TX"; masterrx "LPI2C_MASTER_EVENT_RX"; masterfifoerr "LPI2C_MASTER_EVENT_FIFO_ERROR"; masterarblost "LPI2C_MASTER_EVENT_ARBITRATION_LOST"; masternack "LPI2C_MASTER_EVENT_NACK"
      mask help: This block allows to create routine for the LPI2C interrupts.
      mask init:
      | st = mbd_s32k_lpi2c_isr_tostring();
      | mbd_s32k_lpi2c_display_instances();
      settings: NameChangeFcn=mbd_s32k_name_check(gcb);
      mask Help: web(fullfile(mbd_s32k_block_help, 'lpi2c', 'lpi2c_isr.html'));
      mask TypeOptions instance: 0 | 1
      mask Callback instance: mbd_s32k_lpi2c_display_instances();
      mask TypeOptions mode: Master | Slave
      mask Callback mode: mbd_s32k_lpi2c_isr_mode_ckb(gcb);
      mask Display:
      | disp(st);
      | port_label('output', 1, 'Trigger');
      | image('nxp_logo.png', 'top-right');
  LPI2C_ISR_Disable_Enable : S-Function  FunctionName=lpi2c_s32k_disen  SFunctionDeploymentMode=off  EnableBusSupport=off  mask(lpi2c_s32k_disen){instance=0, master_eot_event=off, m_rdie=off, m_epie=off, m_sdie=off, m_ndie=off, m_alie=off, m_feie=off, s_tdie=off, s_rdie=off, s_rsie=off, s_sdie=off, s_beie=off, s_feie=off, upd=1}
      mask prompts: master_eot_event "Master end of transfer"; m_rdie "Receive Data"; m_epie "End Packet"; m_sdie "STOP Detect"; m_ndie "NACK Detect"; m_alie "Arbitration Lost"; m_feie "FIFO Error"; s_tdie "Transmit Data"; s_rdie "Receive Data"; s_rsie "Repeated Start"; s_sdie "STOP Detect"; s_beie "Bit Error"; s_feie "FIFO Error"
      mask help: This block allows to Enable\Disable I2C ISR routine.
      mask init:
      | mbd_s32k_lpi2c_display_interrupts();
      | mbd_s32k_lpi2c_display_instances();
      | 
      | eol = sprintf('\n');
      | st = ['LPI2C', get_param(gcb, 'instance')];
      | fields = get_param(gcb, 'MaskPrompts');
      | vis = get_param(gcb, 'MaskVisibilities');
      | vals = get_param(gcb, 'MaskValues');
      | 
      | for i = 2 : length(fields) - 1
      |     if (strcmp(vis{i}, 'on'))
      |         s = [eol, fields{i}, ': ', vals{i}];
      |         st = [st, s];
      |     end
      | end
      settings: NameChangeFcn=mbd_s32k_name_check(gcb);
      mask Help: web(fullfile(mbd_s32k_block_help, 'lpi2c', 'lpi2c_disen.html'));
      mask TypeOptions instance: 0 | 1
      mask Callback instance: mbd_s32k_lpi2c_display_instances();
      mask Display:
      | disp(st);
      | image('nxp_logo.png', 'top-right');
  LPI2C_Master_Receive : S-Function  FunctionName=lpi2c_s32k_master_receive  SFunctionDeploymentMode=off  EnableBusSupport=off  mask(lpi2c_s32k_master_receive){instance=0, xfermode=Blocking, Timeout=50, is10bit=off}
      mask prompts: xfermode "Transfer mode"; Timeout "Timeout (ms)"; is10bit "10-bit address"
      mask help: This block allows the master to request data from slave.
      mask init:
      | maskStr = 'LPI2C Master Receive';
      | mbd_s32k_lpi2c_display_instances();
      settings: NameChangeFcn=mbd_s32k_name_check(gcb);
      mask Help: web(fullfile(mbd_s32k_block_help, 'lpi2c', 'lpi2c_master_receive.html'));
      mask TypeOptions instance: 0 | 1
      mask Callback instance: mbd_s32k_lpi2c_display_instances();
      mask TypeOptions xfermode: Blocking | Non blocking
      mask Callback xfermode: mbd_s32k_lpi2c_xfer_mode_cbk()
      mask Display:
      | port_label('output', 1, 'Data');
      | port_label('input', 1, 'Address');
      | port_label('input', 2, 'SendStop');
      | port_label('input', 3, 'Length');
      | disp(maskStr);
      | image('nxp_logo.png', 'top-right');
  LPI2C_Master_Transmit : S-Function  FunctionName=lpi2c_s32k_master_transmit  SFunctionDeploymentMode=off  EnableBusSupport=off  mask(lpi2c_s32k_master_transmit){instance=0, xfermode=Blocking, Timeout=50, is10bit=off}
      mask prompts: xfermode "Transfer mode"; Timeout "Timeout (ms)"; is10bit "10-bit address"
      mask help: This block allows the master to transmit data to the slave.
      mask init:
      | maskStr = 'LPI2C Master Transmit';
      | mbd_s32k_lpi2c_display_instances();
      settings: NameChangeFcn=mbd_s32k_name_check(gcb);
      mask Help: web(fullfile(mbd_s32k_block_help, 'lpi2c', 'lpi2c_master_transmit.html'));
      mask TypeOptions instance: 0 | 1
      mask Callback instance: mbd_s32k_lpi2c_display_instances();
      mask TypeOptions xfermode: Blocking | Non blocking
      mask Callback xfermode: mbd_s32k_lpi2c_xfer_mode_cbk()
      mask Display:
      | port_label('input', 1, 'Data');
      | port_label('input', 2, 'SendStop');
      | port_label('input', 3, 'Address');
      | disp(maskStr);
      | image('nxp_logo.png', 'top-right');
  LPI2C_Slave_Receive : S-Function  FunctionName=lpi2c_s32k_slave_receive  SFunctionDeploymentMode=off  EnableBusSupport=off  mask(lpi2c_s32k_slave_receive){instance=0, xfermode=Blocking, Timeout=50, is10bit=off}
      mask prompts: xfermode "Transfer mode"; Timeout "Timeout (ms)"; is10bit "10-bit address"
      mask help: This block allows the slave to receive data from master.
      mask init:
      | maskStr = 'LPI2C Slave Receive';
      | mbd_s32k_lpi2c_display_instances();
      settings: NameChangeFcn=mbd_s32k_name_check(gcb);
      mask Help: web(fullfile(mbd_s32k_block_help, 'lpi2c', 'lpi2c_slave_receive.html'));
      mask TypeOptions instance: 0 | 1
      mask Callback instance: mbd_s32k_lpi2c_display_instances();
      mask TypeOptions xfermode: Blocking | Non blocking
      mask Callback xfermode: mbd_s32k_lpi2c_xfer_mode_cbk()
      mask Display:
      | port_label('output', 1, 'Data');
      | port_label('input', 1, 'Address');
      | port_label('input', 2, 'Length');
      | disp(maskStr);
      | image('nxp_logo.png', 'top-right');
  LPI2C_Slave_Transmit : S-Function  FunctionName=lpi2c_s32k_slave_transmit  SFunctionDeploymentMode=off  EnableBusSupport=off  mask(lpi2c_s32k_slave_transmit){instance=0, xfermode=Blocking, Timeout=50, is10bit=off}
      mask prompts: xfermode "Transfer mode"; Timeout "Timeout (ms)"; is10bit "10-bit address"
      mask help: This block allows the slave to respond to master request for data.
      mask init:
      | maskStr = 'LPI2C Slave Transmit';
      | mbd_s32k_lpi2c_display_instances();
      settings: NameChangeFcn=mbd_s32k_name_check(gcb);
      mask Help: web(fullfile(mbd_s32k_block_help, 'lpi2c', 'lpi2c_slave_transmit.html'));
      mask TypeOptions instance: 0 | 1
      mask Callback instance: mbd_s32k_lpi2c_display_instances();
      mask TypeOptions xfermode: Blocking | Non blocking
      mask Callback xfermode: mbd_s32k_lpi2c_xfer_mode_cbk()
      mask Display:
      | port_label('input', 1, 'Data');
      | port_label('input', 2, 'Address');
      | disp(maskStr);
      | image('nxp_logo.png', 'top-right');
